simulink model "cross_vzmac_core"  (Simulink 7.9)
settings: Solver=ode45  StartTime=0.0  StopTime=2048*16+100  RelTol=1e-3
PreLoadFcn:
  | if ~exist('sync')
  |   sync=[1];
  | end
  | if ~exist('zin0')
  |   zin0=complex( ...
  |     floor(256*rand(1,15*2048+1))/128-1, ...
  |     floor(256*rand(1,15*2048+1))/128-1  ...
  |   );
  | end
  | if ~exist('zin1')
  |   zin1=complex( ...
  |     floor(256*rand(1,15*2048+1))/128-1, ...
  |     floor(256*rand(1,15*2048+1))/128-1  ...
  |   );
  | end
undefined symbols (not defined in the file or in its folder): A, B, PCIN, xlipgetpartsetting
libraries: xbsIndex_r4 x34
(part 3 of 6)

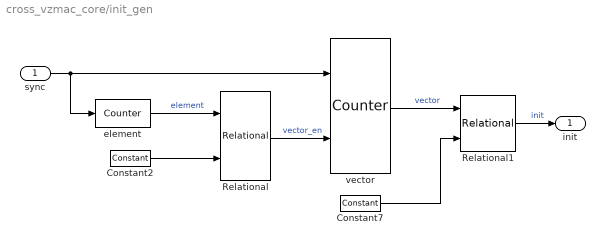
== system cross_vzmac_core/init_gen ==
  sync : Inport
  Constant2 : xbsIndex_r4/Constant  const=2048-2  gui_display_data_type=Fixed-point  arith_type=Unsigned  n_bits=11  bin_pt=0  preci_type=Single  exp_width=8  frac_width=24  explicit_period=on  period=1  equ=P=C  opselect=C  inp2=PCIN>>17  opr=+  inp1=P  carry=CIN  dbl_ovrd=off  block_type=constant
  Constant7 : xbsIndex_r4/Constant  const=0  gui_display_data_type=Fixed-point  arith_type=Unsigned  n_bits=4  bin_pt=0  preci_type=Single  exp_width=8  frac_width=24  explicit_period=on  period=1  equ=P=C  opselect=C  inp2=PCIN>>17  opr=+  inp1=P  carry=CIN  dbl_ovrd=off  block_type=constant
  Relational : xbsIndex_r4/Relational  mode=a=b  en=off  latency=1  dbl_ovrd=off  block_type=relational
  Relational1 : xbsIndex_r4/Relational  mode=a=b  en=off  latency=0  dbl_ovrd=off  block_type=relational
  element : xbsIndex_r4/Counter  cnt_type=Free Running  cnt_to=Inf  operation=Up  start_count=0  cnt_by_val=1  arith_type=Unsigned  n_bits=11  bin_pt=0  load_pin=off  rst=on  en=off  explicit_period=on  period=1  dbl_ovrd=off  use_behavioral_HDL=on  implementation=Fabric  block_type=counter
  vector : xbsIndex_r4/Counter  cnt_type=Count Limited  cnt_to=13  operation=Up  start_count=0  cnt_by_val=1  arith_type=Unsigned  n_bits=4  bin_pt=0  load_pin=off  rst=on  en=on  explicit_period=on  period=1  dbl_ovrd=off  use_behavioral_HDL=on  implementation=Fabric  block_type=counter
  init : Outport
  wires:
  vector/1 -> Relational1/1  "vector"
  Constant7/1 -> Relational1/2
  Constant2/1 -> Relational/2
  Relational/1 -> vector/2  "vector_en"
  element/1 -> Relational/1  "element"
  sync/1 -> vector/1, element/1
  Relational1/1 -> init/1  "init"
